simulink model "power_thyristor"  (Simulink 6.0)
settings: Solver=ode23tb  SolverMode=SingleTasking  StartTime=0.0  StopTime=0.1  RelTol=1e-3
libraries: powerlib x8
settings Model: Creator=patrice  LastModifiedBy=batserve  ExtModeTrigMode=oneshot  ExtModeArmWhenConnect=off  ExtModeAutoUpdateStatusClock=off
settings DataIOCC: LimitDataPoints=off  SaveOutput=off  TimeSaveName=t  SignalLoggingName=sigsOut
settings OptimizationCC: BooleanDataType=off
settings DebuggingCC: SolverPrmCheckMsg=none  UnconnectedInputMsg=none  UnconnectedOutputMsg=none
settings HardwareCC: TargetUnknown=on
settings RTWCC: TemplateMakefile=grt_unix.tmf

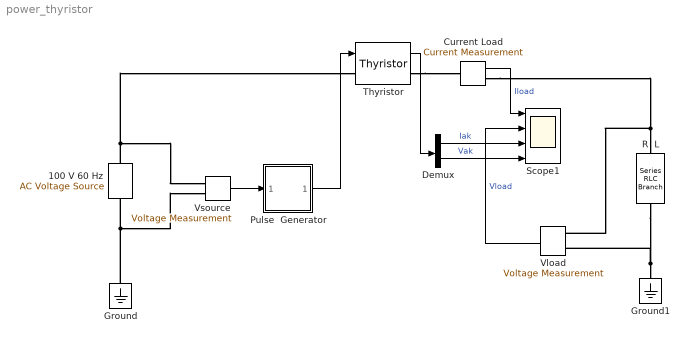
== system power_thyristor ==
  " Pulse  Generator" : Subsystem
      mask Display: plot(0,0,100,100,[90,75,75,60,60,35,35,20,20,10],[20,20,80,80,20,20,80,80,20,20])
  100 V 60 Hz : powerlib/Electrical Sources/AC Voltage Source  Description=source block  Orientation=up  Amplitude=100  Phase=0  Frequency=60  SampleTime=0  Measurements=None
      settings: AttributesFormatString=\n
  Current Load : powerlib/Measurements/Current Measurement  Tag=PoWeRsYsTeMmEaSuReMeNt  PhasorSimulation=off  OutputType=Magnitude  PSBequivalent=0
  Demux : Demux  Outputs=2
  Ground : powerlib/Elements/Ground  Orientation=down  PhysicalDomain=powersysdomain  SubClassName=unknown  PortType=p1  LConnTagsString=a
  Ground1 : powerlib/Elements/Ground  Orientation=down  PhysicalDomain=powersysdomain  SubClassName=unknown  PortType=p1  LConnTagsString=a
  R  L : powerlib/Elements/Series RLC Branch  Orientation=down  PhysicalDomain=powersysdomain  SubClassName=unknown  PortType=p1  LConnTagsString=__new0  RConnTagsString=__new0  Resistance=1  Inductance=10e-03  Capacitance=inf  Measurements=None
  Scope1 : Scope  NumInputPorts=4
      settings: TimeRange=0.1  YMin=-50~-100~0~-200  YMax=50~100~40~200  DataFormat=Array
  Thyristor : powerlib/Power Electronics/Thyristor  Ron=1e-3  Lon=0  Vf=0.8  IC=0  Rs=20  Cs=4e-6  Measurements=on
      settings: AttributesFormatString=\n
  Vload : powerlib/Measurements/Voltage Measurement  Tag=PoWeRsYsTeMmEaSuReMeNt  Orientation=left  PhasorSimulation=off  OutputType=Magnitude  PSBequivalent=0
  Vsource : powerlib/Measurements/Voltage Measurement  Tag=PoWeRsYsTeMmEaSuReMeNt  PhasorSimulation=off  OutputType=Magnitude  PSBequivalent=0
  wires:
  Demux/1 -> Scope1/3  "Iak"
  Demux/2 -> Scope1/4  "Vak"
  Thyristor/1 -> Demux/1
  Current Load/1 -> Scope1/1  "Iload"
  Vload/1 -> Scope1/2  "Vload"
  " Pulse  Generator"/1(out_1) -> Thyristor/1
  Vsource/1 -> " Pulse  Generator"/1(in_1)
  connections:
  Thyristor/RConn1 -- Current Load/LConn1
  Current Load/RConn1 -- Vload/LConn1 -- R  L/LConn1
  Ground1/LConn1 -- R  L/RConn1 -- Vload/LConn2
  Ground/LConn1 -- Vsource/LConn2 -- 100 V 60 Hz/LConn1
  100 V 60 Hz/RConn1 -- Vsource/LConn1 -- Thyristor/LConn1

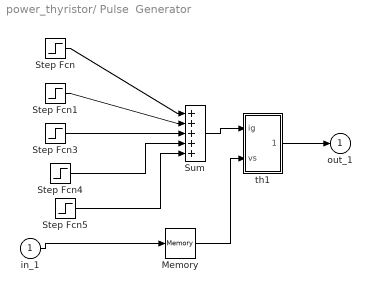
== system power_thyristor/ Pulse  Generator ==
  in_1 : Inport  Port=1  LatchInput=off
  Memory : Memory
  Step Fcn : Step  Time=1/60  Before=20  After=20  SampleTime=0
  Step Fcn1 : Step  Time=1/60  After=30  SampleTime=0
  Step Fcn3 : Step  Time=2/60  After=30  SampleTime=0
  Step Fcn4 : Step  Time=3/60  After=30  SampleTime=0
  Step Fcn5 : Step  Time=4/60  After=30  SampleTime=0
  Sum : Sum  Inputs=+++++  SaturateOnIntegerOverflow=on  InputSameDT=on
  th1 : Subsystem
  out_1 : Outport  InitialOutput=0
  wires:
  th1/1(out_1) -> out_1/1
  Step Fcn/1 -> Sum/1
  Step Fcn1/1 -> Sum/2
  Step Fcn3/1 -> Sum/3
  Step Fcn4/1 -> Sum/4
  Step Fcn5/1 -> Sum/5
  Sum/1 -> th1/1(ig)
  in_1/1 -> Memory/1
  Memory/1 -> th1/2(vs)

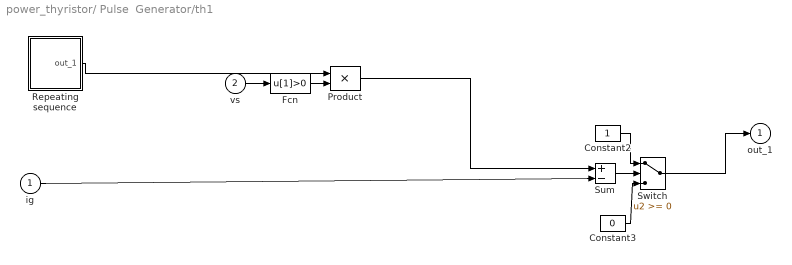
== system power_thyristor/ Pulse  Generator/th1 ==
  ig : Inport  Port=1  LatchInput=off
  vs : Inport  Port=2  LatchInput=off
  Constant2 : Constant
  Constant3 : Constant  Value=0
  Fcn : Fcn  Expr=u[1]>0
  Product : Product  SaturateOnIntegerOverflow=on  InputSameDT=on
  Repeating sequence : Subsystem  mask(Repeating table){@1=[0 1/60 ], @2=[0 360 ]}
      mask prompts: @1 "Time values:"; @2 "Output values:"
      mask help:
      | Repeating table.
      | Enter values of time and output for first cycle.
      mask init:
      | period = max(@1); t = @1; y = @2;
      mask Help: Repeats cycle given in table. Time values should be monotonically increasing.
      mask Display: plot([t,t+period,t+2*period],[y,y,y])
  Sum : Sum  Inputs=+-  SaturateOnIntegerOverflow=on  InputSameDT=on
  Switch : Switch  SaturateOnIntegerOverflow=on  InputSameDT=on
  out_1 : Outport  InitialOutput=0
  wires:
  Product/1 -> Sum/1
  vs/1 -> Fcn/1
  Fcn/1 -> Product/2
  Repeating sequence/1(out_1) -> Product/1
  ig/1 -> Sum/2
  Constant3/1 -> Switch/3
  Constant2/1 -> Switch/1
  Sum/1 -> Switch/2
  Switch/1 -> out_1/1

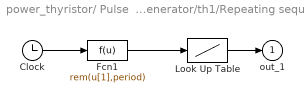
== system power_thyristor/ Pulse  Generator/th1/Repeating sequence ==
  Clock : Clock
      settings: Decimation=10
  Fcn1 : Fcn  Expr=rem(u[1],period)
  Look Up Table : Lookup  DialogController=Simulink.DDGSource  InputValues=t  OutputValues=y  SaturateOnIntegerOverflow=on
  out_1 : Outport  InitialOutput=0
  wires:
  Fcn1/1 -> Look Up Table/1
  Clock/1 -> Fcn1/1
  Look Up Table/1 -> out_1/1
